simulink library "Wind_env"  (R2018b)
settings: Solver=VariableStepAuto  StartTime=0.0  StopTime=10.0  RelTol=1e-3
values from neighbouring files (symbols this model uses):
  r = 4    [glob.m]
undefined symbols (not defined in the file or in its folder): F, magnitude, MIL, rate_x, rate_y, rate_z, xwind_l, xwind_u, ywind_l, ywind_u, zwind_l, zwind_u
libraries: aerolibwind2 x3, simulink x3, sharedtransform x1
settings Model: Creator=Andrew Garcia  LastModifiedBy=Andrew Garcia

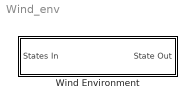
== system Wind_env ==
  "Wind Environment " : Subsystem  LoadFcn=big_pam  InitFcn=big_pam

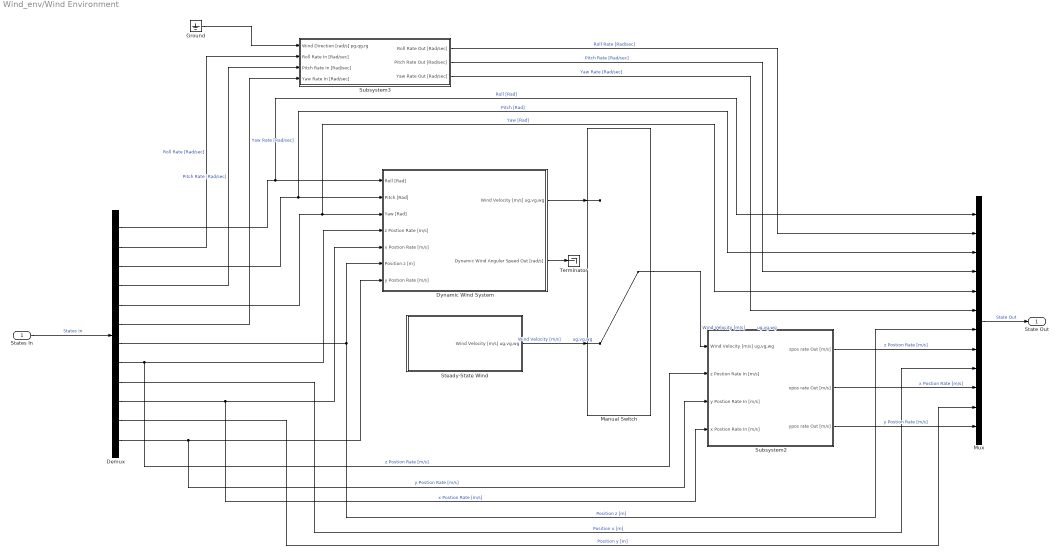
== system Wind_env/Wind Environment  ==
  States In : Inport
  Demux : Demux  Outputs=12
  Dynamic Wind System : Subsystem
  Ground : Ground
  Manual Switch : ManualSwitch  CurrentSetting=0
  Mux : Mux  Inputs=12
  Steady-State Wind : Subsystem
  Subsystem2 : Subsystem
  Subsystem3 : Subsystem
  Terminator : Terminator
  State Out : Outport
  wires:
  Mux/1 -> State Out/1  "State Out"
  Dynamic Wind System/2(Dynamic Wind Anguler Speed Out [rad/s]) -> Terminator/1
  Dynamic Wind System/1(Wind Velocity [m/s] ug,vg,wg) -> Manual Switch/1
  Demux/12 -> Subsystem2/3(y Postion Rate In [m/s]), Dynamic Wind System/7(y Postion Rate [m/s])  "y Postion Rate [m/s]"
  Demux/10 -> Subsystem2/4(x Postion Rate In [m/s]), Dynamic Wind System/5(x Postion Rate [m/s])  "x Postion Rate [m/s]"
  Demux/8 -> Subsystem2/2(z Postion Rate In [m/s]), Dynamic Wind System/4(z Postion Rate [m/s])  "z Postion Rate [m/s]"
  Ground/1 -> Subsystem3/1(Wind Direction [rad/s] pg,qg,rg)
  Subsystem2/3(ypos rate Out [m/s]) -> Mux/12  "y Postion Rate [m/s]"
  Demux/11 -> Mux/11  "Position y [m]"
  Subsystem2/2(xpos rate Out [m/s]) -> Mux/10  "x Postion Rate [m/s]"
  Subsystem2/1(zpos rate Out [m/s]) -> Mux/8  "z Postion Rate [m/s]"
  Subsystem3/3(Yaw Rate Out [Rad/sec]) -> Mux/6  "Yaw Rate [Rad/sec]"
  Demux/5 -> Mux/5, Dynamic Wind System/3(Yaw [Rad])  "Yaw [Rad]"
  Subsystem3/2(Pitch Rate Out [Rad/sec]) -> Mux/4  "Pitch Rate [Rad/sec]"
  Demux/3 -> Mux/3, Dynamic Wind System/2(Pitch [Rad])  "Pitch [Rad]"
  Subsystem3/1(Roll Rate Out [Rad/sec]) -> Mux/2  "Roll Rate [Rad/sec]"
  Demux/1 -> Mux/1, Dynamic Wind System/1(Roll [Rad])  "Roll [Rad]"
  States In/1 -> Demux/1  "States In"
  Demux/9 -> Mux/9  "Position x [m]"
  Demux/7 -> Mux/7, Dynamic Wind System/6(Position z [m])  "Position z [m]"
  Demux/2 -> Subsystem3/2(Roll Rate In [Rad/sec])  "Roll Rate [Rad/sec]"
  Demux/6 -> Subsystem3/4(Yaw Rate In [Rad/sec])  "Yaw Rate [Rad/sec]"
  Demux/4 -> Subsystem3/3(Pitch Rate In [Rad/sec])  "Pitch Rate [Rad/sec]"
  Manual Switch/1 -> Subsystem2/1(Wind Velocity [m/s] ug,vg,wg)  "Wind Velocity [m/s]         ug,vg,wg"
  Steady-State Wind/1(Wind Velocity [m/s] ug,vg,wg) -> Manual Switch/2  "Wind Velocity [m/s]         ug,vg,wg"

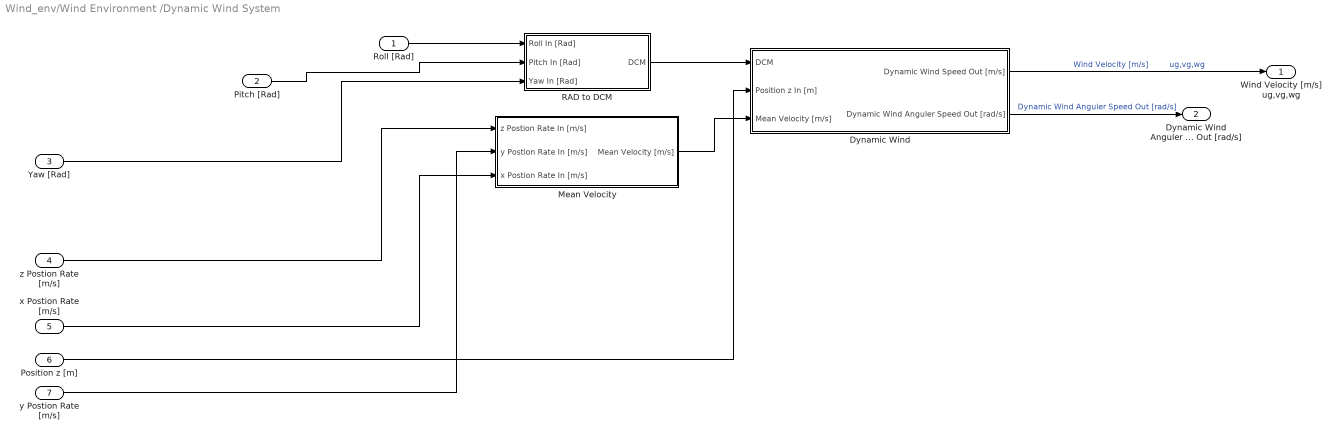
== system Wind_env/Wind Environment /Dynamic Wind System ==
  Roll [Rad] : Inport
  Pitch [Rad] : Inport  Port=2
  Yaw [Rad] : Inport  Port=3
  z Postion Rate [m/s] : Inport  Port=4
  x Postion Rate [m/s] : Inport  Port=5
  Position z [m] : Inport  Port=6
  y Postion Rate [m/s] : Inport  Port=7
  Dynamic Wind : Subsystem
  "Mean Velocity " : Subsystem
  RAD to DCM : Subsystem
  Wind Velocity [m/s] ug,vg,wg : Outport
  Dynamic Wind Anguler Speed Out [rad/s] : Outport  Port=2
  wires:
  Yaw [Rad]/1 -> RAD to DCM/3(Yaw In [Rad])
  Roll [Rad]/1 -> RAD to DCM/1(Roll In [Rad])
  Dynamic Wind/1(Dynamic Wind Speed Out [m/s]) -> Wind Velocity [m/s] ug,vg,wg/1  "Wind Velocity [m/s]         ug,vg,wg"
  x Postion Rate [m/s]/1 -> "Mean Velocity "/3(x Postion Rate In [m/s])
  y Postion Rate [m/s]/1 -> "Mean Velocity "/2(y Postion Rate In [m/s])
  Pitch [Rad]/1 -> RAD to DCM/2(Pitch In [Rad])
  Position z [m]/1 -> Dynamic Wind/2(Position z In [m])
  Dynamic Wind/2(Dynamic Wind Anguler Speed Out [rad/s]) -> Dynamic Wind Anguler Speed Out [rad/s]/1  "Dynamic Wind Anguler Speed Out [rad/s]"
  "Mean Velocity "/1(Mean Velocity [m/s]) -> Dynamic Wind/3(Mean Velocity [m/s])
  z Postion Rate [m/s]/1 -> "Mean Velocity "/1(z Postion Rate In [m/s])
  RAD to DCM/1(DCM) -> Dynamic Wind/1(DCM)

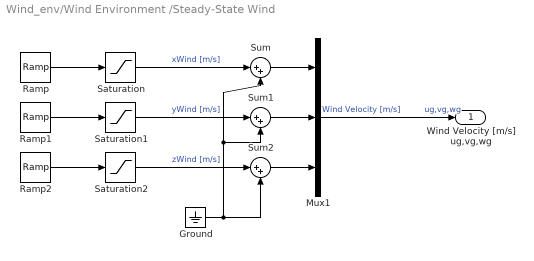
== system Wind_env/Wind Environment /Steady-State Wind ==
  Ground : Ground
  Mux1 : Mux  Inputs=3
  Ramp : simulink/Sources/Ramp  slope=rate_x  start=0  InitialOutput=0
  Ramp1 : simulink/Sources/Ramp  slope=rate_y  start=0  InitialOutput=0
  Ramp2 : simulink/Sources/Ramp  slope=rate_z  start=0  InitialOutput=0
  Saturation : Saturate  UpperLimit=xwind_u  LowerLimit=xwind_l
  Saturation1 : Saturate  UpperLimit=ywind_u  LowerLimit=ywind_l
  Saturation2 : Saturate  UpperLimit=zwind_u  LowerLimit=zwind_l
  Sum : Sum  Inputs=|++
  Sum1 : Sum  Inputs=|++
  Sum2 : Sum  Inputs=|++
  Wind Velocity [m/s] ug,vg,wg : Outport
  wires:
  Ramp2/1 -> Saturation2/1
  Ramp1/1 -> Saturation1/1
  Ramp/1 -> Saturation/1
  Ground/1 -> Sum2/2, Sum1/2, Sum/2
  Sum2/1 -> Mux1/3
  Sum1/1 -> Mux1/2
  Sum/1 -> Mux1/1
  Saturation2/1 -> Sum2/1  "zWind [m/s]"
  Saturation1/1 -> Sum1/1  "yWind [m/s]"
  Saturation/1 -> Sum/1  "xWind [m/s]"
  Mux1/1 -> Wind Velocity [m/s] ug,vg,wg/1  "Wind Velocity [m/s]         ug,vg,wg"

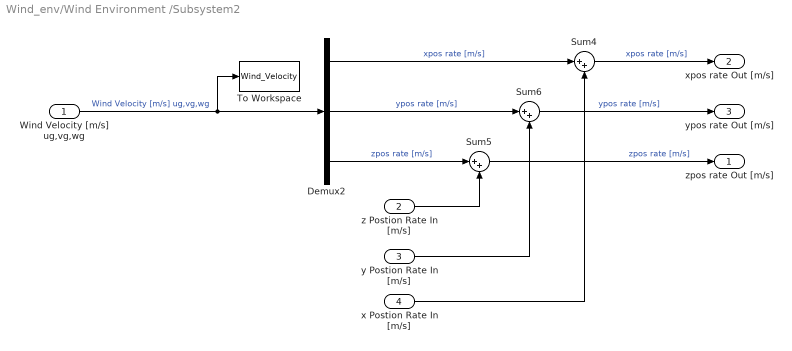
== system Wind_env/Wind Environment /Subsystem2 ==
  Wind Velocity [m/s] ug,vg,wg : Inport
  z Postion Rate In [m/s] : Inport  Port=2
  y Postion Rate In [m/s] : Inport  Port=3
  x Postion Rate In [m/s] : Inport  Port=4
  Demux2 : Demux  Outputs=3
  Sum4 : Sum  Inputs=|++
  Sum5 : Sum  Inputs=|++
  Sum6 : Sum  Inputs=|++
  To Workspace : ToWorkspace  VariableName=Wind_Velocity  SaveFormat=Timeseries  SampleTime=-1
  zpos rate Out [m/s] : Outport
  xpos rate Out [m/s] : Outport  Port=2
  ypos rate Out [m/s] : Outport  Port=3
  wires:
  Sum4/1 -> xpos rate Out [m/s]/1  "xpos rate [m/s]"
  z Postion Rate In [m/s]/1 -> Sum5/2
  Sum5/1 -> zpos rate Out [m/s]/1  "zpos rate [m/s]"
  Demux2/2 -> Sum6/1  "ypos rate [m/s]"
  x Postion Rate In [m/s]/1 -> Sum4/2
  y Postion Rate In [m/s]/1 -> Sum6/2
  Sum6/1 -> ypos rate Out [m/s]/1  "ypos rate [m/s]"
  Demux2/3 -> Sum5/1  "zpos rate [m/s]"
  Wind Velocity [m/s] ug,vg,wg/1 -> Demux2/1, To Workspace/1  "Wind Velocity [m/s] ug,vg,wg"
  Demux2/1 -> Sum4/1  "xpos rate [m/s]"

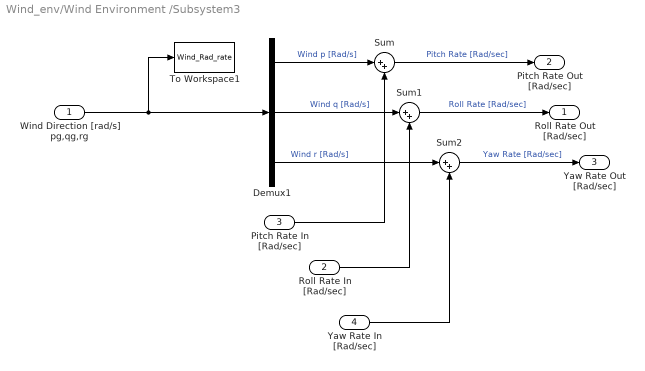
== system Wind_env/Wind Environment /Subsystem3 ==
  Wind Direction [rad/s] pg,qg,rg : Inport
  Roll Rate In [Rad/sec] : Inport  Port=2
  Pitch Rate In [Rad/sec] : Inport  Port=3
  Yaw Rate In [Rad/sec] : Inport  Port=4
  Demux1 : Demux  Outputs=3
  Sum : Sum  Inputs=|++
  Sum1 : Sum  Inputs=|++
  Sum2 : Sum  Inputs=|++
  To Workspace1 : ToWorkspace  VariableName=Wind_Rad_rate  SaveFormat=Timeseries  SampleTime=-1
  Roll Rate Out [Rad/sec] : Outport
  Pitch Rate Out [Rad/sec] : Outport  Port=2
  Yaw Rate Out [Rad/sec] : Outport  Port=3
  wires:
  Sum1/1 -> Roll Rate Out [Rad/sec]/1  "Roll Rate [Rad/sec]"
  Roll Rate In [Rad/sec]/1 -> Sum1/2
  Demux1/3 -> Sum2/1  "Wind r [Rad/s]"
  Wind Direction [rad/s] pg,qg,rg/1 -> Demux1/1, To Workspace1/1
  Yaw Rate In [Rad/sec]/1 -> Sum2/2
  Sum/1 -> Pitch Rate Out [Rad/sec]/1  "Pitch Rate [Rad/sec]"
  Pitch Rate In [Rad/sec]/1 -> Sum/2
  Sum2/1 -> Yaw Rate Out [Rad/sec]/1  "Yaw Rate [Rad/sec]"
  Demux1/2 -> Sum1/1  "Wind q [Rad/s]"
  Demux1/1 -> Sum/1  "Wind p [Rad/s]"

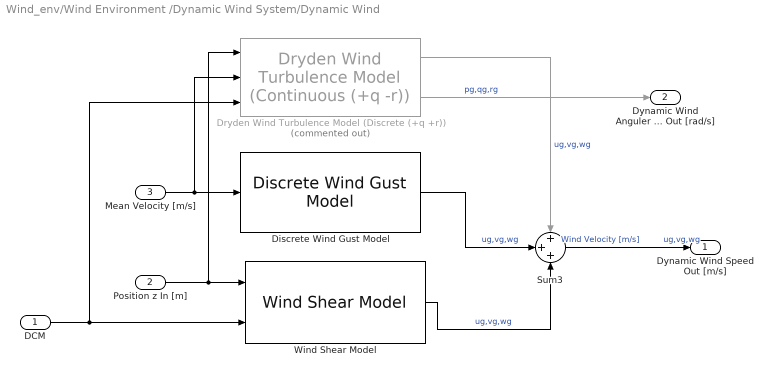
== system Wind_env/Wind Environment /Dynamic Wind System/Dynamic Wind ==
  DCM : Inport
  Position z In [m] : Inport  Port=2
  Mean Velocity [m/s] : Inport  Port=3
  Discrete Wind Gust Model : aerolibwind2/Discrete Wind Gust Model  units=Metric (MKS)  Gx=on  Gy=on  Gz=on  t_0=5  d_m=[30 30 20]  v_m=[2.5 2.5 2.0]
      settings: SourceProductName=Aerospace Blockset
  Dryden Wind Turbulence Model (Discrete (+q +r)) : aerolibwind2/Dryden Wind Turbulence Model  (Continuous (+q -r))  Commented=on  units=Metric (MKS)  spec=MIL-F-8785C  model=Discrete Dryden (+q +r)  W20=3  Wdeg=0  TurbProb=2x10^-1  L_high=10  Wingspan=.2  ts=0.1  Seed=[324 234 2342 232]  T_on=on
      settings: SourceProductName=Aerospace Blockset
  Sum3 : Sum  Inputs=+++
  Wind Shear Model : aerolibwind2/Wind Shear Model  units=Metric (MKS)  phase=Other  W_20=2  Wdeg=0
      settings: SourceProductName=Aerospace Blockset
  Dynamic Wind Speed Out [m/s] : Outport
  Dynamic Wind Anguler Speed Out [rad/s] : Outport  Port=2
  wires:
  Dryden Wind Turbulence Model (Discrete (+q +r))/1 -> Sum3/1  "ug,vg,wg"
  Discrete Wind Gust Model/1 -> Sum3/2  "ug,vg,wg"
  DCM/1 -> Dryden Wind Turbulence Model (Discrete (+q +r))/3, Wind Shear Model/2
  Position z In [m]/1 -> Wind Shear Model/1, Dryden Wind Turbulence Model (Discrete (+q +r))/1
  Sum3/1 -> Dynamic Wind Speed Out [m/s]/1  "Wind Velocity [m/s]         ug,vg,wg"
  Wind Shear Model/1 -> Sum3/3  "ug,vg,wg"
  Mean Velocity [m/s]/1 -> Discrete Wind Gust Model/1, Dryden Wind Turbulence Model (Discrete (+q +r))/2
  Dryden Wind Turbulence Model (Discrete (+q +r))/2 -> Dynamic Wind Anguler Speed Out [rad/s]/1  "pg,qg,rg"

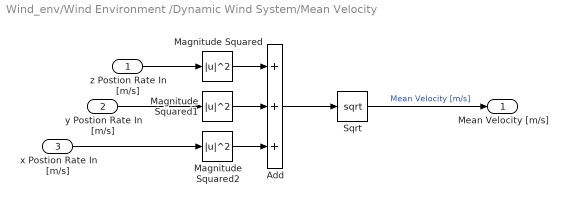
== system Wind_env/Wind Environment /Dynamic Wind System/Mean Velocity  ==
  z Postion Rate In [m/s] : Inport
  y Postion Rate In [m/s] : Inport  Port=2
  x Postion Rate In [m/s] : Inport  Port=3
  Add : Sum  Inputs=+++
  Magnitude Squared : Math  Operator=magnitude^2  SaturateOnIntegerOverflow=on
  Magnitude Squared1 : Math  Operator=magnitude^2  SaturateOnIntegerOverflow=on
  Magnitude Squared2 : Math  Operator=magnitude^2  SaturateOnIntegerOverflow=on
  Sqrt : Sqrt  SaturateOnIntegerOverflow=on
  Mean Velocity [m/s] : Outport
  wires:
  y Postion Rate In [m/s]/1 -> Magnitude Squared1/1
  Add/1 -> Sqrt/1
  x Postion Rate In [m/s]/1 -> Magnitude Squared2/1
  Magnitude Squared/1 -> Add/1
  Magnitude Squared1/1 -> Add/2
  Magnitude Squared2/1 -> Add/3
  Sqrt/1 -> Mean Velocity [m/s]/1  "Mean Velocity [m/s]"
  z Postion Rate In [m/s]/1 -> Magnitude Squared/1

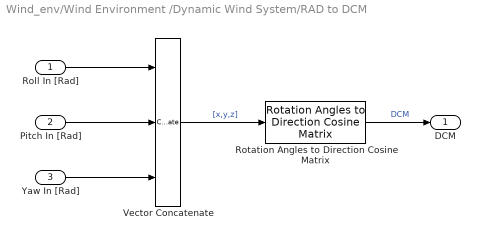
== system Wind_env/Wind Environment /Dynamic Wind System/RAD to DCM ==
  Roll In [Rad] : Inport
  Pitch In [Rad] : Inport  Port=2
  Yaw In [Rad] : Inport  Port=3
  Rotation Angles to Direction Cosine Matrix : sharedtransform/Rotation Angles to Direction Cosine Matrix  rotationOrder=XYZ  aMode=aMode
      settings: SourceProductBaseCode=AE
  Vector Concatenate : Concatenate  NumInputs=3
  DCM : Outport
  wires:
  Roll In [Rad]/1 -> Vector Concatenate/1
  Pitch In [Rad]/1 -> Vector Concatenate/2
  Yaw In [Rad]/1 -> Vector Concatenate/3
  Rotation Angles to Direction Cosine Matrix/1 -> DCM/1  "DCM"
  Vector Concatenate/1 -> Rotation Angles to Direction Cosine Matrix/1  "[x,y,z]"
